simulink model "tensegrity_Val_like_sim_one_stage_v02"  (R2022b)
settings: Solver=ode15s  StartTime=0.0  StopTime=10  MaxStep=0.001  RelTol=1e-3
InitFcn:
  | tensegrity_Val_like_v02;
values from neighbouring files (symbols this model uses):
  a = 0.015    [parameters.m]
  A1 = [0.3, 0.3, 0.2]    [parameters_test_model.m]    (also in tensegrity_Val_like.m = [(G1+G2+G3)/3])
  A2 = [(G4+G5+G6)/3]    [tensegrity_Val_like.m]
  A3 = [(G7+G8+G9)/3]    [tensegrity_Val_like.m]
  A4 = [(B1+B2+B3)/3]    [tensegrity_Val_like.m]
  b_all = 2*ones(6, 1)    [parameters_test_model.m]
  F1 = [pos1(1), pos1(2), pos1(3)]    [parameters.m]
  F2 = [pos1(1)+dist, pos1(2), pos1(3)]    [parameters.m]
  F3 = [pos1(1)+dist/2, pos1(2)+dist, pos1(3)]    [parameters.m]
  F4 = [pos2(1), pos2(2), pos2(3)]    [parameters.m]
  F5 = [pos2(1)+dist, pos2(2), pos2(3)]    [parameters.m]
  F6 = [pos2(1)+dist/2, pos2(2)+dist, pos2(3)]    [parameters.m]
  F7 = [pos3(1), pos3(2), pos3(3)]    [parameters.m]
  F8 = [pos3(1)+dist, pos3(2), pos3(3)]    [parameters.m]
  F9 = [pos3(1)+dist/2, pos3(2)+dist, pos3(3)]    [parameters.m]
  k_all = 1e3*ones(6, 1)    [parameters_test_model.m]
  l = [0.08 0.08 0.08 0.15]'    [parameters.m]
  l0_all = [l01, l02, l03, l04, l05, l06]'    [parameters_test_model.m]
  lf = 0.05*ones(9, 1)    [parameters.m]
  predpeti = 0.95    [parameters_test_model.m]
undefined symbols (not defined in the file or in its folder): X, Y, Z
libraries: sm_lib x76, nesl_utility x73
(part 4 of 4)

== matlab function tensegrity_Val_like_sim_one_stage_v02/internal cable force_13/cable force/parameter selection/parameter selection ==
  data: i input; k output; k_all input; b_all input; l0_all input; b output; l0 output
function [k, b, l0] = parameter_selection(i, k_all, b_all, l0_all)

k=k_all(i);
b=b_all(i);
l0=l0_all(i);

== matlab function tensegrity_Val_like_sim_one_stage_v02/internal cable force_120/cable force/cable force computation ==
  data: k input; Fc output; b input; l0 input; l input; v input
function Fc = cable_force(k, b,l0, l, v)

Fc=k*(l-l0) + b*v;

== matlab function tensegrity_Val_like_sim_one_stage_v02/internal cable force_120/cable force/parameter selection/parameter selection ==
  data: i input; k output; k_all input; b_all input; l0_all input; b output; l0 output
function [k, b, l0] = parameter_selection(i, k_all, b_all, l0_all)

k=k_all(i);
b=b_all(i);
l0=l0_all(i);

== matlab function tensegrity_Val_like_sim_one_stage_v02/internal cable force_19/cable force/cable force computation ==
  data: k input; Fc output; b input; l0 input; l input; v input
function Fc = cable_force(k, b,l0, l, v)

Fc=k*(l-l0) + b*v;

== matlab function tensegrity_Val_like_sim_one_stage_v02/internal cable force_19/cable force/parameter selection/parameter selection ==
  data: i input; k output; k_all input; b_all input; l0_all input; b output; l0 output
function [k, b, l0] = parameter_selection(i, k_all, b_all, l0_all)

k=k_all(i);
b=b_all(i);
l0=l0_all(i);

== matlab function tensegrity_Val_like_sim_one_stage_v02/internal cable force_3/cable force/cable force computation ==
  data: k input; Fc output; b input; l0 input; l input; v input
function Fc = cable_force(k, b,l0, l, v)

Fc=k*(l-l0) + b*v;

== matlab function tensegrity_Val_like_sim_one_stage_v02/internal cable force_16/cable force/cable force computation ==
  data: k input; Fc output; b input; l0 input; l input; v input
function Fc = cable_force(k, b,l0, l, v)

Fc=k*(l-l0) + b*v;

== matlab function tensegrity_Val_like_sim_one_stage_v02/internal cable force_16/cable force/parameter selection/parameter selection ==
  data: i input; k output; k_all input; b_all input; l0_all input; b output; l0 output
function [k, b, l0] = parameter_selection(i, k_all, b_all, l0_all)

k=k_all(i);
b=b_all(i);
l0=l0_all(i);

== matlab function tensegrity_Val_like_sim_one_stage_v02/internal cable force_14/cable force/cable force computation ==
  data: k input; Fc output; b input; l0 input; l input; v input
function Fc = cable_force(k, b,l0, l, v)

Fc=k*(l-l0) + b*v;

== matlab function tensegrity_Val_like_sim_one_stage_v02/internal cable force_14/cable force/parameter selection/parameter selection ==
  data: i input; k output; k_all input; b_all input; l0_all input; b output; l0 output
function [k, b, l0] = parameter_selection(i, k_all, b_all, l0_all)

k=k_all(i);
b=b_all(i);
l0=l0_all(i);

== matlab function tensegrity_Val_like_sim_one_stage_v02/internal cable force_15/cable force/cable force computation ==
  data: k input; Fc output; b input; l0 input; l input; v input
function Fc = cable_force(k, b,l0, l, v)

Fc=k*(l-l0) + b*v;

== matlab function tensegrity_Val_like_sim_one_stage_v02/internal cable force_15/cable force/parameter selection/parameter selection ==
  data: i input; k output; k_all input; b_all input; l0_all input; b output; l0 output
function [k, b, l0] = parameter_selection(i, k_all, b_all, l0_all)

k=k_all(i);
b=b_all(i);
l0=l0_all(i);

== matlab function tensegrity_Val_like_sim_one_stage_v02/internal cable force_17/cable force/cable force computation ==
  data: k input; Fc output; b input; l0 input; l input; v input
function Fc = cable_force(k, b,l0, l, v)

Fc=k*(l-l0) + b*v;

== matlab function tensegrity_Val_like_sim_one_stage_v02/internal cable force_17/cable force/parameter selection/parameter selection ==
  data: i input; k output; k_all input; b_all input; l0_all input; b output; l0 output
function [k, b, l0] = parameter_selection(i, k_all, b_all, l0_all)

k=k_all(i);
b=b_all(i);
l0=l0_all(i);

== matlab function tensegrity_Val_like_sim_one_stage_v02/internal cable force_18/cable force/cable force computation ==
  data: k input; Fc output; b input; l0 input; l input; v input
function Fc = cable_force(k, b,l0, l, v)

Fc=k*(l-l0) + b*v;

== matlab function tensegrity_Val_like_sim_one_stage_v02/internal cable force_3/cable force/parameter selection/parameter selection ==
  data: i input; k output; k_all input; b_all input; l0_all input; b output; l0 output
function [k, b, l0] = parameter_selection(i, k_all, b_all, l0_all)

k=k_all(i);
b=b_all(i);
l0=l0_all(i);

== matlab function tensegrity_Val_like_sim_one_stage_v02/internal cable force_18/cable force/parameter selection/parameter selection ==
  data: i input; k output; k_all input; b_all input; l0_all input; b output; l0 output
function [k, b, l0] = parameter_selection(i, k_all, b_all, l0_all)

k=k_all(i);
b=b_all(i);
l0=l0_all(i);

== matlab function tensegrity_Val_like_sim_one_stage_v02/internal cable force_20/cable force/cable force computation ==
  data: k input; Fc output; b input; l0 input; l input; v input
function Fc = cable_force(k, b,l0, l, v)

Fc=k*(l-l0) + b*v;

== matlab function tensegrity_Val_like_sim_one_stage_v02/internal cable force_20/cable force/parameter selection/parameter selection ==
  data: i input; k output; k_all input; b_all input; l0_all input; b output; l0 output
function [k, b, l0] = parameter_selection(i, k_all, b_all, l0_all)

k=k_all(i);
b=b_all(i);
l0=l0_all(i);

== matlab function tensegrity_Val_like_sim_one_stage_v02/internal cable force_21/cable force/cable force computation ==
  data: k input; Fc output; b input; l0 input; l input; v input
function Fc = cable_force(k, b,l0, l, v)

Fc=k*(l-l0) + b*v;

== matlab function tensegrity_Val_like_sim_one_stage_v02/internal cable force_21/cable force/parameter selection/parameter selection ==
  data: i input; k output; k_all input; b_all input; l0_all input; b output; l0 output
function [k, b, l0] = parameter_selection(i, k_all, b_all, l0_all)

k=k_all(i);
b=b_all(i);
l0=l0_all(i);

== matlab function tensegrity_Val_like_sim_one_stage_v02/internal cable force_22/cable force/cable force computation ==
  data: k input; Fc output; b input; l0 input; l input; v input
function Fc = cable_force(k, b,l0, l, v)

Fc=k*(l-l0) + b*v;

== matlab function tensegrity_Val_like_sim_one_stage_v02/internal cable force_22/cable force/parameter selection/parameter selection ==
  data: i input; k output; k_all input; b_all input; l0_all input; b output; l0 output
function [k, b, l0] = parameter_selection(i, k_all, b_all, l0_all)

k=k_all(i);
b=b_all(i);
l0=l0_all(i);

== matlab function tensegrity_Val_like_sim_one_stage_v02/internal cable force_23/cable force/cable force computation ==
  data: k input; Fc output; b input; l0 input; l input; v input
function Fc = cable_force(k, b,l0, l, v)

Fc=k*(l-l0) + b*v;

== matlab function tensegrity_Val_like_sim_one_stage_v02/internal cable force_23/cable force/parameter selection/parameter selection ==
  data: i input; k output; k_all input; b_all input; l0_all input; b output; l0 output
function [k, b, l0] = parameter_selection(i, k_all, b_all, l0_all)

k=k_all(i);
b=b_all(i);
l0=l0_all(i);

== matlab function tensegrity_Val_like_sim_one_stage_v02/internal cable force_4/cable force/cable force computation ==
  data: k input; Fc output; b input; l0 input; l input; v input
function Fc = cable_force(k, b,l0, l, v)

Fc=k*(l-l0) + b*v;

== matlab function tensegrity_Val_like_sim_one_stage_v02/internal cable force_4/cable force/parameter selection/parameter selection ==
  data: i input; k output; k_all input; b_all input; l0_all input; b output; l0 output
function [k, b, l0] = parameter_selection(i, k_all, b_all, l0_all)

k=k_all(i);
b=b_all(i);
l0=l0_all(i);

== matlab function tensegrity_Val_like_sim_one_stage_v02/internal cable force_5/cable force/cable force computation ==
  data: k input; Fc output; b input; l0 input; l input; v input
function Fc = cable_force(k, b,l0, l, v)

Fc=k*(l-l0) + b*v;

== matlab function tensegrity_Val_like_sim_one_stage_v02/internal cable force_5/cable force/parameter selection/parameter selection ==
  data: i input; k output; k_all input; b_all input; l0_all input; b output; l0 output
function [k, b, l0] = parameter_selection(i, k_all, b_all, l0_all)

k=k_all(i);
b=b_all(i);
l0=l0_all(i);
